simulink model "Tachometer_Sim"  (R2017a)
settings: Solver=FixedStepDiscrete  StartTime=0.0  StopTime=inf  FixedStep=0.005  RelTol=1e-3  EnableMultiTasking=on
undefined symbols (not defined in the file): fdesignblkfcn, gcbh
libraries: dsparch4 x1
settings Model: ExtModeTrigDuration=5000  Creator=Admin  LastModifiedBy=cchan
settings SolverCC: PositivePriorityOrder=on
settings DataIOCC: LimitDataPoints=on  SaveFormat=Array  SignalLoggingSaveFormat=ModelDataLogs
settings OptimizationCC: ExpressionDepthLimit=2147483647  LifeSpan=inf
settings DebuggingCC: UnderspecifiedInitializationDetection=Classic  MergeDetectMultiDrivingBlocksExec=none  SolverPrmCheckMsg=warning  FcnCallInpInsideContextMsg=warning  AllowSymbolicDim=off  StateNameClashWarn=warning  SFUnexpectedBacktrackingDiag=warning  SFNoUnconditionalDefaultTransitionDiag=warning  SFExecutionAtInitializationDiag=none
settings HardwareCC: ProdBitPerPointer=32  ProdBitPerSizeT=32  ProdBitPerPtrDiffT=32  ProdLargestAtomicFloat=None  ProdIntDivRoundTo=Undefined  ProdEndianess=Unspecified  ProdWordSize=32  ProdHWDeviceType=32-bit Generic
settings ModelReferenceCC: PropagateSignalLabelsOutOfModel=off
settings RTWCC: SystemTargetFile=quarc_win64.tlc  TemplateMakefile=quarc_default_tmf  Description=QUARC Win64 Target
settings STFCustomTargetCC: TargetPreCompLibLocation=C:\PROGRA~3\QUARC\lib\2015b\win64\release  ConcurrentExecutionCompliant=on  SystemTargetFile=quarc_win64.tlc
settings GRTTargetCC: TargetPreCompLibLocation=C:\PROGRA~3\QUARC\lib\2015b\win64\release  TargetLangStandard=C89/C90 (ANSI)  ParMdlRefBuildCompliant=off  CompOptLevelCompliant=off  CombineOutputUpdateFcns=off  MatFileLogging=off  CPPClassGenCompliant=off  GRTInterface=on  UseToolchainInfoCompliant=off  ExtMode=on  ExtModeMexFile=quarc_comm
settings ConfigComp: CovMetricSettings=dw  CovHtmlReporting=on  CovSaveCumulativeToWorkspaceVar=on  CovSaveSingleToWorkspaceVar=on  CovExternalEMLEnable=off

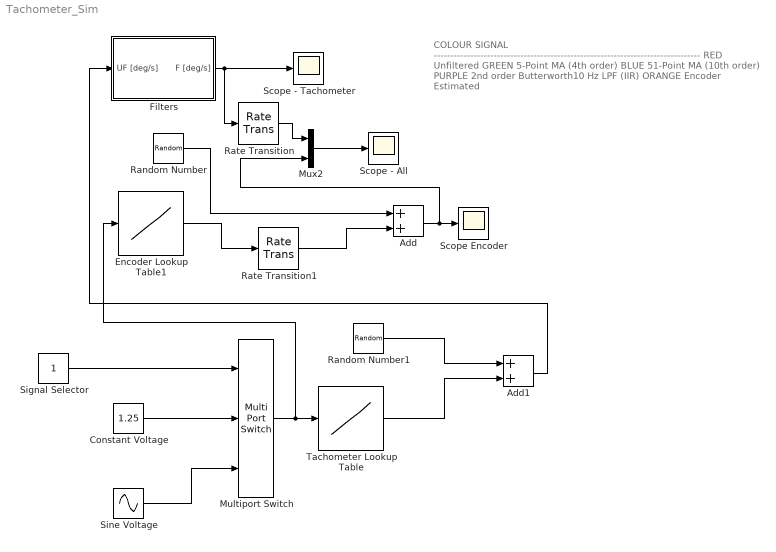
== system Tachometer_Sim ==
  note: COLOUR SIGNAL
      | --------------------------------------------------------------------------------
      | RED Unfiltered
      | GREEN 5-Point MA (4th order)
      | BLUE 51-Point MA (10th order)
      | PURPLE 2nd order Butterworth10 Hz LPF (IIR)
      | ORANGE Encoder Estimated
  Add : Sum
  Add1 : Sum
  Constant Voltage : Constant  Value=1.25
  Encoder Lookup Table1 : Lookup_n-D  NumberOfTableDimensions=1  BreakpointsForDimension1=[-3:1:3]  Table=[-265, -171, -78, 0, 81, 176, 275]  InternalRulePriority=Speed  RndMeth=Simplest  InputSameDT=on
  Filters : Subsystem
  Multiport Switch : MultiPortSwitch  Inputs=2
  Mux2 : Mux  Inputs=2
  Random Number : RandomNumber  Variance=1.5  SampleTime=0.02
  Random Number1 : RandomNumber  Variance=6.5  SampleTime=0.1
  Rate Transition : RateTransition  OutPortSampleTime=0.02
  Rate Transition1 : RateTransition  OutPortSampleTime=0.02
  Scope Encoder : Scope
  "Scope - All " : Scope
  Scope - Tachometer : Scope
  Signal Selector : Constant
  Sine Voltage : Sin  Amplitude=.25  Bias=1  Frequency=2*pi  SampleTime=0.1
  Tachometer Lookup Table : Lookup_n-D  NumberOfTableDimensions=1  BreakpointsForDimension1=[-5:1:5]  Table=[-502,-397.9,-293.5,-190.9,-87.95,0,92.42,194.3,295.4,398.6,502.7]  InternalRulePriority=Speed  RndMeth=Simplest  InputSameDT=on
  wires:
  Filters/1(F [deg/s]) -> Rate Transition/1, Scope - Tachometer/1
  Mux2/1 -> "Scope - All "/1
  Signal Selector/1 -> Multiport Switch/1
  Sine Voltage/1 -> Multiport Switch/3
  Constant Voltage/1 -> Multiport Switch/2
  Multiport Switch/1 -> Encoder Lookup Table1/1, Tachometer Lookup Table/1
  Random Number/1 -> Add/1
  Add/1 -> Mux2/2, Scope Encoder/1
  Random Number1/1 -> Add1/1
  Add1/1 -> Filters/1(UF [deg/s])
  Encoder Lookup Table1/1 -> Rate Transition1/1
  Rate Transition1/1 -> Add/2
  Tachometer Lookup Table/1 -> Add1/2
  Rate Transition/1 -> Mux2/1

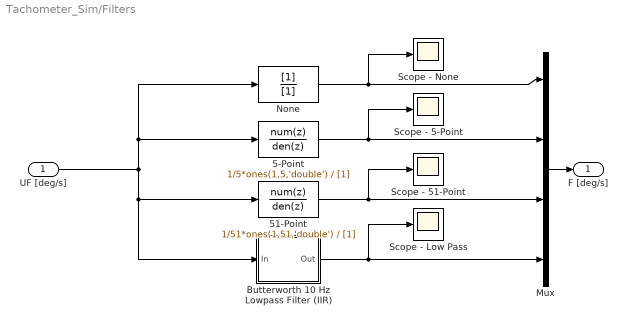
== system Tachometer_Sim/Filters ==
  UF [deg/s] : Inport
  5-Point : DiscreteFilter  Numerator=1/5*ones(1,5,'double')  Denominator=[1]
  51-Point : DiscreteFilter  Numerator=1/51*ones(1,51,'double')  Denominator=[1]
  Butterworth 10 Hz Lowpass Filter (IIR) : Subsystem  DialogController=fdesignblkfcn  InitFcn=fdesignblkfcn(gcbh, {'InitFcn'});  mask(Lowpass Filter){}
      mask help: Design a lowpass filter
      settings: CopyFcn=fdesignblkfcn(gcbh, {'CopyFcn'});
      mask Help: helpview(mapfilelocation('dsp'), 'dsplowpassfilter');
      mask Display: disp('Lowpass')
  Mux : Mux
  None : DiscreteFilter  Denominator=[1]
  Scope - 5-Point : Scope
  Scope - 51-Point : Scope
  Scope - Low Pass : Scope
  Scope - None : Scope
  F [deg/s] : Outport
  wires:
  Butterworth 10 Hz Lowpass Filter (IIR)/1(Out) -> Mux/4, Scope - Low Pass/1
  51-Point/1 -> Mux/3, Scope - 51-Point/1
  5-Point/1 -> Mux/2, Scope - 5-Point/1
  None/1 -> Mux/1, Scope - None/1
  UF [deg/s]/1 -> 51-Point/1, Butterworth 10 Hz Lowpass Filter (IIR)/1(In), None/1, 5-Point/1
  Mux/1 -> F [deg/s]/1

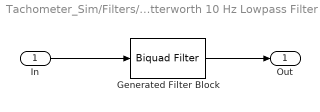
== system Tachometer_Sim/Filters/Butterworth 10 Hz Lowpass Filter (IIR) ==
  In : Inport
  Generated Filter Block : dsparch4/Biquad Filter  Tag=BlockMethodSubSystem  IIRFiltStruct=Direct form II  CoeffSource=Specify via dialog  BiQuadCoeffs=[0.250078647993701 0.500157295987402 0.250078647993701 1 -1.5610180758007179 0.64135153805756318]  a0Flag=Warning  IC=0  ICnum=0  ICden=0  InputProcessing=Columns as channels (frame based)  denAccumFracLength=30  denProdOutputFracLength=30  secondMemoryFracLength=15  roundingMode=Floor  overflowMode=off  ScaleValues=[0.080308197942261336;1]  optimizeScaleValues=off  ScaleValueMode=Specify via input port (g)  scaleValueFracLength=14  FilterSource=Specify via dialog  FilterObject=BQF
      settings: SourceProductName=DSP System Toolbox
  Out : Outport
  wires:
  In/1 -> Generated Filter Block/1
  Generated Filter Block/1 -> Out/1
